simulink model "VOC7"  (R2022b)
settings: Solver=VariableStepAuto  StartTime=0.0  StopTime=2  RelTol=1e-3
libraries: spsIGBTDiodeLib x12, spsSeriesRLCBranchLib x7, eeRmsMeasurement x6, spsVoltageMeasurementLib x4, spsCurrentMeasurementLib x3, spsDCVoltageSourceLib x3, spspowerguiLib x1
settings Model: Creator=LEGION  LastModifiedBy=DoCongHieu
settings DebuggingCC: UnconnectedInputMsg=warning  UnconnectedOutputMsg=warning  UnconnectedLineMsg=warning
settings ModelReferenceCC: EnableRefExpFcnMdlSchedulingChecks=on
settings RTWCC: DLArmComputeVersion=19.05

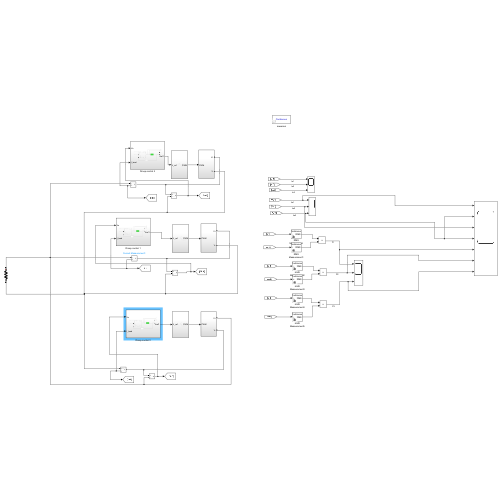
[thumbnail: Simulink's stored preview of the top-level diagram]
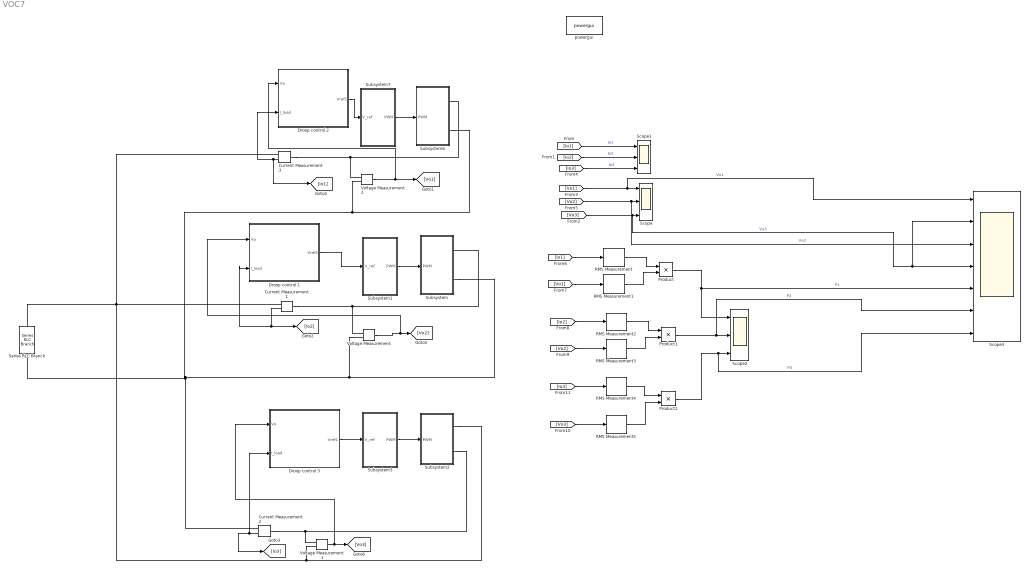
== system VOC7 ==
  Current Measurement1 : spsCurrentMeasurementLib/Current Measurement  PhasorSimulation=off  OutputType=Complex  PSBequivalent=0
  Current Measurement2 : spsCurrentMeasurementLib/Current Measurement  PhasorSimulation=off  OutputType=Complex  PSBequivalent=0
  Current Measurement3 : spsCurrentMeasurementLib/Current Measurement  PhasorSimulation=off  OutputType=Complex  PSBequivalent=0
  Droop control 1 : Subsystem
  Droop control 2 : Subsystem
  Droop control 3 : Subsystem
  Product : Product
  Product1 : Product
  Product2 : Product
  RMS Measurement{,1..5} (6 alike) : eeRmsMeasurement/RMS Measurement  LabelModeActiveChoice=Total  F=60  SpecifyHarmonics=off  K=[0 1 2]  Ts=0
      settings: LibrarySourceBlock=|
      | ee_sl_lib/Measurements/RMS
      | Measurement
  Scope : Scope  NumInputPorts=3
  Scope1 : Scope  NumInputPorts=3
  Scope2 : Scope  NumInputPorts=3
  Scope3 : Scope  NumInputPorts=7
  Series RLC Branch : spsSeriesRLCBranchLib/Series RLC Branch  LConnTagsString=__new0  RConnTagsString=__new0  BranchType=R  Resistance=10  Inductance=1e-3  SetiL0=off  InitialCurrent=0  Capacitance=1e-6  Setx0=off  InitialVoltage=0  Measurements=None
  Subsystem : Subsystem
  Subsystem1 : Subsystem
  Subsystem2 : Subsystem
  Subsystem3 : Subsystem
  Subsystem6 : Subsystem
  Subsystem7 : Subsystem
  Voltage Measurement : spsVoltageMeasurementLib/Voltage Measurement  PhasorSimulation=off  OutputType=Complex  PSBequivalent=0
  Voltage Measurement1 : spsVoltageMeasurementLib/Voltage Measurement  PhasorSimulation=off  OutputType=Complex  PSBequivalent=0
  Voltage Measurement2 : spsVoltageMeasurementLib/Voltage Measurement  PhasorSimulation=off  OutputType=Complex  PSBequivalent=0
  powergui : spspowerguiLib/powergui  Priority=1  SimulationMode=Continuous  SampleTime=5e-6  frequency=60  Iterations=50  frequencyindice=0  Pbase=100e6  ErrMax=1e-4  UnitsV=kV  UnitsW=MW  buscounter=0  FunctionMessages=off  echomessages=off  EnableUseOfTLC=off  CurrentSourceSwitches=off  DisableSnubberDevices=off  DisableRonSwitches=off  DisableVfSwitches=off  DisplayEquations=off  AutomaticDiscreteSolvers=off  SolverType=Tustin/Backward Euler (TBE)  Interpol=off  ExternalGateDelay=off  methode=off  Ts=100  x0status=blocks  SPID=on  SwTol=0  HookPort=off  NonlinearTolerance=1e-4  nMaxIteration=100  ContinueOnMaxIteration=off  RestoreLinks=warning  ResistiveCurrentMeasurement=off  Frange=[0:2:500]  Ylog=off  Xlog=on  ShowGrid=off  save=off  variable=ZData  structure=0  ZoomFFT=off  StartTime=0.0  cycles=1  DisplayStyle=1  fundamental=60  FreqAxis=off  MaxFrequency=1000  frequencyindicesteady=1  RmsSteady=1  display=off
  wires:
  Current Measurement1/1 -> [Io2], Droop control 1/2(I_load)
  [Io2] -> Scope1/2  "Io2"
  [Io1] -> Scope1/1  "Io1"
  Subsystem1/1(PWM) -> Subsystem/1(PWM)
  Subsystem3/1(PWM) -> Subsystem2/1("PWM ")
  RMS Measurement/1 -> Product/1
  RMS Measurement1/1 -> Product/2
  Voltage Measurement/1 -> Droop control 1/1(Vo), [Vo2]
  [Vo1] -> Scope3/1, Scope/1  "Vo1"
  [Vo2] -> Scope3/3, Scope/2  "Vo2"
  [Vo1] -> RMS Measurement1/1
  [Io1] -> RMS Measurement/1
  RMS Measurement3/1 -> Product1/2
  [Vo2] -> RMS Measurement3/1
  [Io2] -> RMS Measurement2/1
  RMS Measurement2/1 -> Product1/1
  Product/1 -> Scope2/1, Scope3/5  "P1"
  Product1/1 -> Scope3/6, Scope2/2  "P2"
  Subsystem7/1(PWM) -> Subsystem6/1(PWM)
  Current Measurement3/1 -> Droop control 2/2(I_load), [Io1]
  Voltage Measurement2/1 -> Droop control 2/1(Vo), [Vo1]
  RMS Measurement5/1 -> Product2/2
  RMS Measurement4/1 -> Product2/1
  Product2/1 -> Scope3/7, Scope2/3  "P3"
  [Vo3] -> Scope3/2, Scope3/4, Scope/3  "Vo3"
  [Io3] -> Scope1/3  "Io3"
  [Vo3] -> RMS Measurement5/1
  [Io3] -> RMS Measurement4/1
  Droop control 1/1(Vref1) -> Subsystem1/1(V_ref)
  Droop control 2/1(Vref1) -> Subsystem7/1(V_ref)
  Voltage Measurement1/1 -> Droop control 3/1(Vo), [Vo3]
  Current Measurement2/1 -> Droop control 3/2(I_load), [Io3]
  Droop control 3/1(Vref1) -> Subsystem3/1(V_ref)
  connections:
  Current Measurement1/LConn1 -- Voltage Measurement/LConn1 -- Subsystem/RConn1
  Series RLC Branch/LConn1 -- Voltage Measurement1/LConn2 -- Subsystem2/RConn1 -- Current Measurement3/RConn1 -- Current Measurement1/RConn1
  Subsystem6/RConn1 -- Current Measurement3/LConn1 -- Voltage Measurement2/LConn1
  Series RLC Branch/RConn1 -- Subsystem/RConn2 -- Voltage Measurement/LConn2 -- Subsystem6/RConn2 -- Voltage Measurement2/LConn2 -- Current Measurement2/RConn1
  Subsystem2/RConn2 -- Voltage Measurement1/LConn1 -- Current Measurement2/LConn1

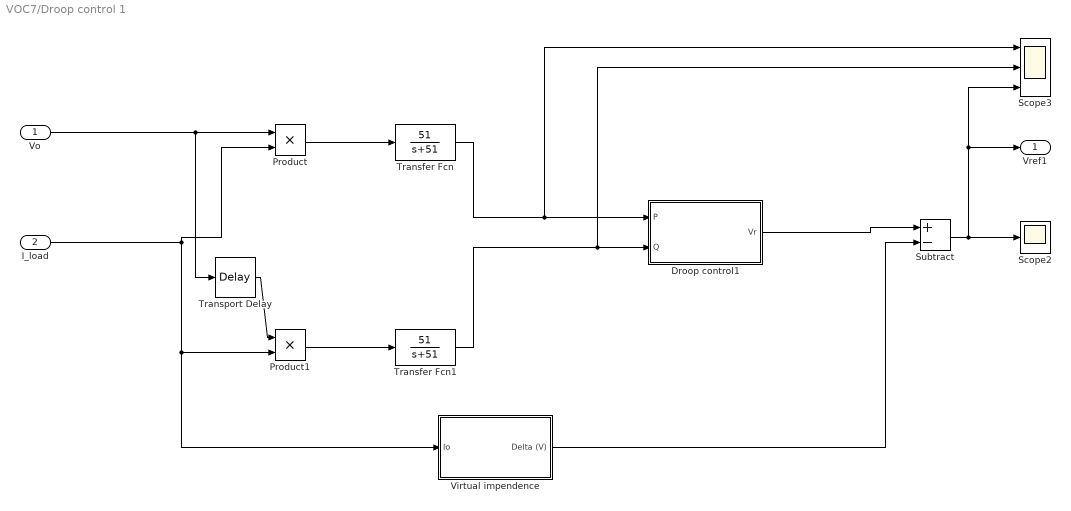
== system VOC7/Droop control 1 ==
  Vo : Inport
  I_load : Inport  Port=2
  Droop control1 : Subsystem  mask{Mi=0.0081, Ni=7.85e-4, E_ref=200*1.1, f_ref=1.01*50, f=50}
      mask prompts: Mi "Vol.coefficient"; Ni "Fre.coefficent"; E_ref "Ref.voltage"; f_ref "Ref.frequency"; f "Fund.frequency"
  Product : Product
  Product1 : Product
  Scope2 : Scope
  Scope3 : Scope  NumInputPorts=3
  Subtract : Sum  Inputs=+-
  Transfer Fcn : TransferFcn  Numerator=[51]  Denominator=[1 51]
  Transfer Fcn1 : TransferFcn  Numerator=[51]  Denominator=[1 51]
  Transport Delay : TransportDelay  DelayTime=0.02/4
  Virtual impendence : Subsystem  mask{fp=150, Rv=0, Lv=2e-3}
      mask prompts: fp "Cutoff Fred"
  Vref1 : Outport
  wires:
  Vo/1 -> Product/1, Transport Delay/1
  I_load/1 -> Product/2, Virtual impendence/1(Io), Product1/2
  Transport Delay/1 -> Product1/1
  Product/1 -> Transfer Fcn/1
  Product1/1 -> Transfer Fcn1/1
  Virtual impendence/1(Delta (V)) -> Subtract/2
  Transfer Fcn1/1 -> Scope3/2, Droop control1/2(Q)
  Droop control1/1(Vr) -> Subtract/1
  Transfer Fcn/1 -> Scope3/1, Droop control1/1(P)
  Subtract/1 -> Scope2/1, Scope3/3, Vref1/1

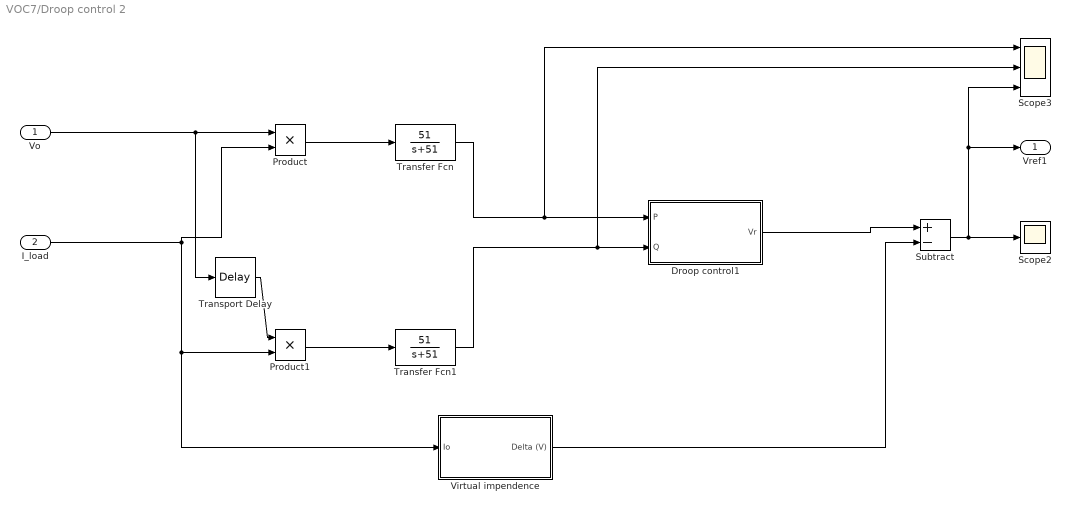
== system VOC7/Droop control 2 ==
  Vo : Inport
  I_load : Inport  Port=2
  Droop control1 : Subsystem  mask{Mi=0.0081, Ni=7.85e-4, E_ref=200*1.1, f_ref=1.01*50, f=50}
      mask prompts: Mi "Vol.coefficient"; Ni "Fre.coefficent"; E_ref "Ref.voltage"; f_ref "Ref.frequency"; f "Fund.frequency"
  Product : Product
  Product1 : Product
  Scope2 : Scope
  Scope3 : Scope  NumInputPorts=3
  Subtract : Sum  Inputs=+-
  Transfer Fcn : TransferFcn  Numerator=[51]  Denominator=[1 51]
  Transfer Fcn1 : TransferFcn  Numerator=[51]  Denominator=[1 51]
  Transport Delay : TransportDelay  DelayTime=0.02/4
  Virtual impendence : Subsystem  mask{fp=150, Rv=0, Lv=2e-3}
      mask prompts: fp "Cutoff Fred"
  Vref1 : Outport
  wires:
  Vo/1 -> Product/1, Transport Delay/1
  I_load/1 -> Product/2, Virtual impendence/1(Io), Product1/2
  Transport Delay/1 -> Product1/1
  Product/1 -> Transfer Fcn/1
  Product1/1 -> Transfer Fcn1/1
  Virtual impendence/1(Delta (V)) -> Subtract/2
  Transfer Fcn1/1 -> Scope3/2, Droop control1/2(Q)
  Droop control1/1(Vr) -> Subtract/1
  Transfer Fcn/1 -> Scope3/1, Droop control1/1(P)
  Subtract/1 -> Scope2/1, Scope3/3, Vref1/1

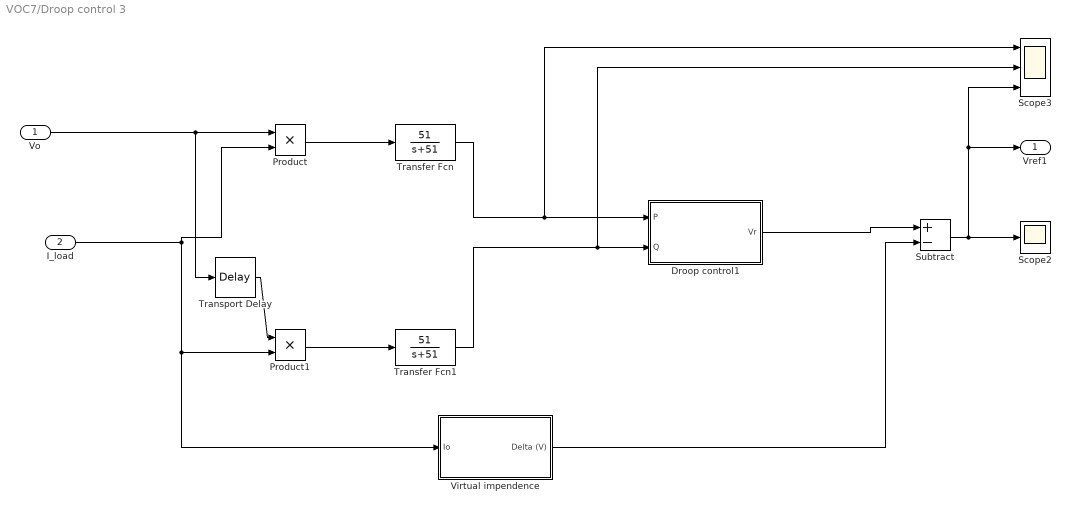
== system VOC7/Droop control 3 ==
  Vo : Inport
  I_load : Inport  Port=2
  Droop control1 : Subsystem  mask{Mi=0.0081, Ni=7.85e-4, E_ref=200*1.1, f_ref=1.01*50, f=50}
      mask prompts: Mi "Vol.coefficient"; Ni "Fre.coefficent"; E_ref "Ref.voltage"; f_ref "Ref.frequency"; f "Fund.frequency"
  Product : Product
  Product1 : Product
  Scope2 : Scope
  Scope3 : Scope  NumInputPorts=3
  Subtract : Sum  Inputs=+-
  Transfer Fcn : TransferFcn  Numerator=[51]  Denominator=[1 51]
  Transfer Fcn1 : TransferFcn  Numerator=[51]  Denominator=[1 51]
  Transport Delay : TransportDelay  DelayTime=0.02/4
  Virtual impendence : Subsystem  mask{fp=150, Rv=0, Lv=2e-3}
      mask prompts: fp "Cutoff Fred"
  Vref1 : Outport
  wires:
  Vo/1 -> Product/1, Transport Delay/1
  I_load/1 -> Product/2, Virtual impendence/1(Io), Product1/2
  Transport Delay/1 -> Product1/1
  Product/1 -> Transfer Fcn/1
  Product1/1 -> Transfer Fcn1/1
  Virtual impendence/1(Delta (V)) -> Subtract/2
  Transfer Fcn1/1 -> Scope3/2, Droop control1/2(Q)
  Droop control1/1(Vr) -> Subtract/1
  Transfer Fcn/1 -> Scope3/1, Droop control1/1(P)
  Subtract/1 -> Scope2/1, Scope3/3, Vref1/1

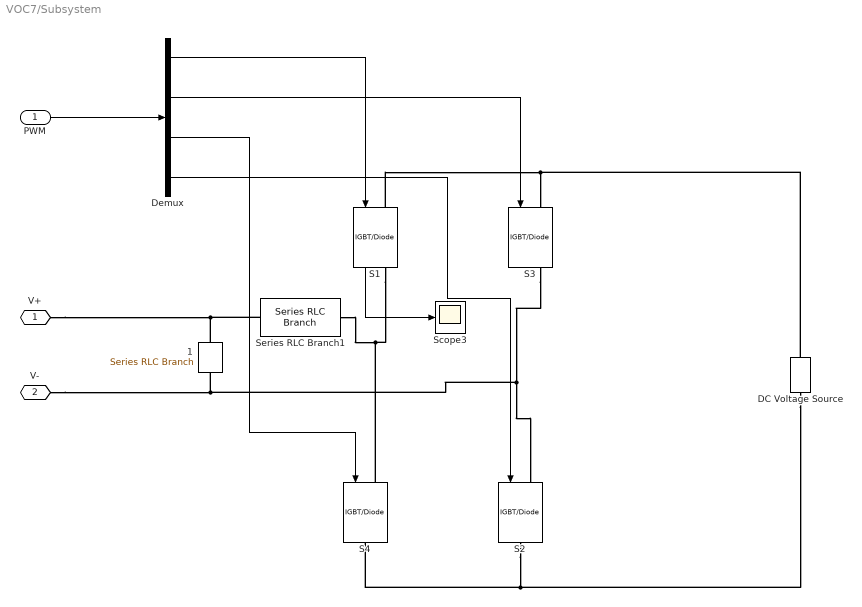
== system VOC7/Subsystem ==
  PWM : Inport
  " 1" : spsSeriesRLCBranchLib/Series RLC Branch  LConnTagsString=__new0  RConnTagsString=__new0  BranchType=C  Resistance=1  Inductance=1e-3  SetiL0=off  InitialCurrent=0  Capacitance=0.00009044  Setx0=off  InitialVoltage=0  Measurements=None
  DC Voltage Source : spsDCVoltageSourceLib/DC Voltage Source  Amplitude=350  Measurements=None
  Demux : Demux
  S1 : spsIGBTDiodeLib/IGBT//Diode  Ron=1e-3  Rs=1e5  Cs=inf  Measurements=on
  S2 : spsIGBTDiodeLib/IGBT//Diode  Ron=1e-3  Rs=1e5  Cs=inf  Measurements=off
  S3 : spsIGBTDiodeLib/IGBT//Diode  Ron=1e-3  Rs=1e5  Cs=inf  Measurements=on
  S4 : spsIGBTDiodeLib/IGBT//Diode  Ron=1e-3  Rs=1e5  Cs=inf  Measurements=off
  Scope3 : Scope
  Series RLC Branch1 : spsSeriesRLCBranchLib/Series RLC Branch  LConnTagsString=__new0  RConnTagsString=__new0  BranchType=L  Resistance=1  Inductance=0.0002882  SetiL0=off  InitialCurrent=0  Capacitance=1e-6  Setx0=off  InitialVoltage=0  Measurements=None
  V+ : PMIOPort  Side=Right
  V- : PMIOPort  Port=2  Side=Right
  wires:
  Demux/1 -> S1/1
  Demux/2 -> S3/1
  Demux/3 -> S4/1
  Demux/4 -> S2/1
  S1/1 -> Scope3/1
  PWM/1 -> Demux/1
  connections:
  DC Voltage Source/RConn1 -- S3/LConn1 -- S1/LConn1
  DC Voltage Source/LConn1 -- S4/RConn1 -- S2/RConn1
  S2/LConn1 -- S3/RConn1 -- V-/RConn1 -- " 1"/RConn1
  S4/LConn1 -- Series RLC Branch1/RConn1 -- S1/RConn1
  V+/RConn1 -- Series RLC Branch1/LConn1 -- " 1"/LConn1

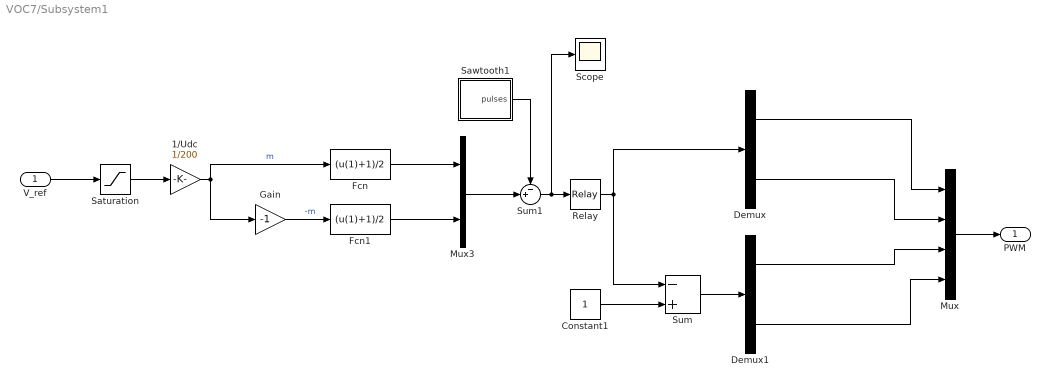
== system VOC7/Subsystem1 ==
  V_ref : Inport
  1/Udc : Gain  Gain=1/200
  Constant1 : Constant
  Demux : Demux  Outputs=2
  Demux1 : Demux  Outputs=2
  Fcn : Fcn  Expr=(u(1)+1)/2
  Fcn1 : Fcn  Expr=(u(1)+1)/2
  Gain : Gain  Gain=-1
  Mux : Mux
  Mux3 : Mux  Inputs=2
  Relay : Relay
  Saturation : Saturate  UpperLimit=310  LowerLimit=-310
  Sawtooth1 : Subsystem
  Scope : Scope
  Sum : Sum  Inputs=-+
  Sum1 : Sum  Inputs=-+|  InputSameDT=on  SaturateOnIntegerOverflow=on  OutDataTypeStr=Inherit: Same as first input
  PWM : Outport
  wires:
  Relay/1 -> Demux/1, Sum/1
  Saturation/1 -> 1/Udc/1
  Demux1/1 -> Mux/3
  Sum/1 -> Demux1/1
  Fcn1/1 -> Mux3/2
  Gain/1 -> Fcn1/1  "-m"
  Constant1/1 -> Sum/2
  1/Udc/1 -> Fcn/1, Gain/1  "m"
  Sum1/1 -> Scope/1, Relay/1
  Demux/2 -> Mux/2
  Demux1/2 -> Mux/4
  Demux/1 -> Mux/1
  Sawtooth1/1(pulses) -> Sum1/1
  Mux3/1 -> Sum1/2
  Fcn/1 -> Mux3/1
  V_ref/1 -> Saturation/1
  Mux/1 -> PWM/1

== system VOC7/Subsystem2 ==
  "PWM " : Inport
  " 1" : spsSeriesRLCBranchLib/Series RLC Branch  LConnTagsString=__new0  RConnTagsString=__new0  BranchType=C  Resistance=1  Inductance=1e-3  SetiL0=off  InitialCurrent=0  Capacitance=0.00009044  Setx0=off  InitialVoltage=0  Measurements=None
  DC Voltage Source : spsDCVoltageSourceLib/DC Voltage Source  Amplitude=350  Measurements=None
  Demux : Demux
  S1 : spsIGBTDiodeLib/IGBT//Diode  Ron=1e-3  Rs=1e5  Cs=inf  Measurements=on
  S2 : spsIGBTDiodeLib/IGBT//Diode  Ron=1e-3  Rs=1e5  Cs=inf  Measurements=off
  S3 : spsIGBTDiodeLib/IGBT//Diode  Ron=1e-3  Rs=1e5  Cs=inf  Measurements=on
  S4 : spsIGBTDiodeLib/IGBT//Diode  Ron=1e-3  Rs=1e5  Cs=inf  Measurements=off
  Series RLC Branch1 : spsSeriesRLCBranchLib/Series RLC Branch  LConnTagsString=__new0  RConnTagsString=__new0  BranchType=L  Resistance=1  Inductance=0.0002882  SetiL0=off  InitialCurrent=0  Capacitance=1e-6  Setx0=off  InitialVoltage=0  Measurements=None
  V+ : PMIOPort  Side=Right
  V- : PMIOPort  Port=2  Side=Right
  wires:
  Demux/1 -> S1/1
  Demux/2 -> S3/1
  Demux/3 -> S4/1
  Demux/4 -> S2/1
  "PWM "/1 -> Demux/1
  connections:
  DC Voltage Source/RConn1 -- S1/LConn1 -- S3/LConn1
  DC Voltage Source/LConn1 -- S4/RConn1 -- S2/RConn1
  S3/RConn1 -- V-/RConn1 -- " 1"/RConn1 -- S2/LConn1
  S4/LConn1 -- S1/RConn1 -- Series RLC Branch1/RConn1
  Series RLC Branch1/LConn1 -- V+/RConn1 -- " 1"/LConn1

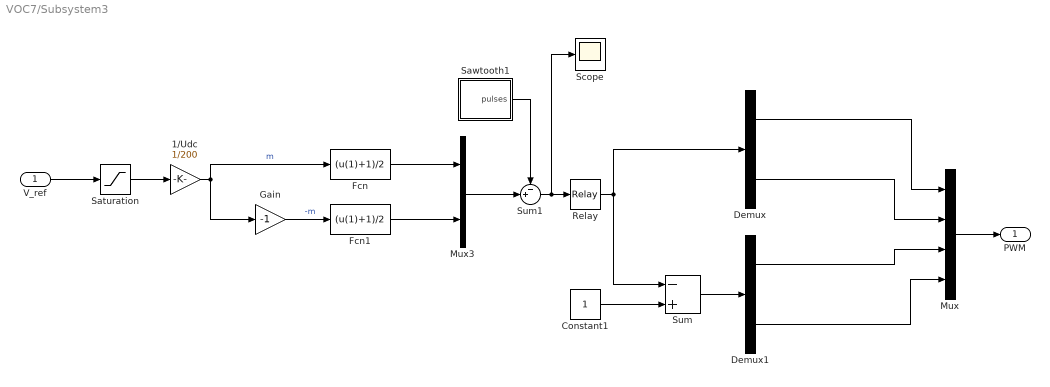
== system VOC7/Subsystem3 ==
  V_ref : Inport
  1/Udc : Gain  Gain=1/200
  Constant1 : Constant
  Demux : Demux  Outputs=2
  Demux1 : Demux  Outputs=2
  Fcn : Fcn  Expr=(u(1)+1)/2
  Fcn1 : Fcn  Expr=(u(1)+1)/2
  Gain : Gain  Gain=-1
  Mux : Mux
  Mux3 : Mux  Inputs=2
  Relay : Relay
  Saturation : Saturate  UpperLimit=310  LowerLimit=-310
  Sawtooth1 : Subsystem
  Scope : Scope
  Sum : Sum  Inputs=-+
  Sum1 : Sum  Inputs=-+|  InputSameDT=on  SaturateOnIntegerOverflow=on  OutDataTypeStr=Inherit: Same as first input
  PWM : Outport
  wires:
  Relay/1 -> Demux/1, Sum/1
  Saturation/1 -> 1/Udc/1
  Demux1/1 -> Mux/3
  Sum/1 -> Demux1/1
  Fcn1/1 -> Mux3/2
  Gain/1 -> Fcn1/1  "-m"
  Constant1/1 -> Sum/2
  1/Udc/1 -> Fcn/1, Gain/1  "m"
  Sum1/1 -> Scope/1, Relay/1
  Demux/2 -> Mux/2
  Demux1/2 -> Mux/4
  Demux/1 -> Mux/1
  Sawtooth1/1(pulses) -> Sum1/1
  Mux3/1 -> Sum1/2
  Fcn/1 -> Mux3/1
  V_ref/1 -> Saturation/1
  Mux/1 -> PWM/1

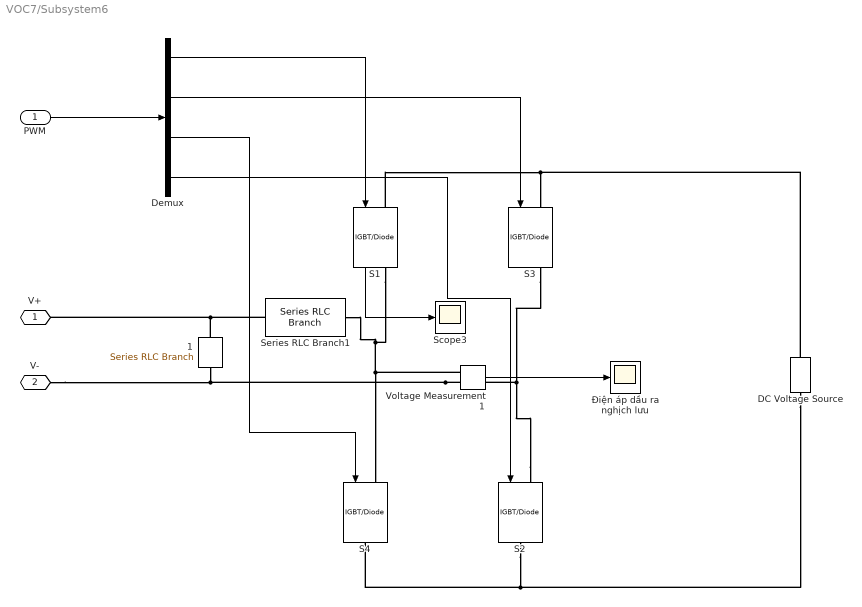
== system VOC7/Subsystem6 ==
  PWM : Inport
  " 1" : spsSeriesRLCBranchLib/Series RLC Branch  LConnTagsString=__new0  RConnTagsString=__new0  BranchType=C  Resistance=1  Inductance=1e-3  SetiL0=off  InitialCurrent=0  Capacitance=0.00009044  Setx0=off  InitialVoltage=0  Measurements=None
  DC Voltage Source : spsDCVoltageSourceLib/DC Voltage Source  Amplitude=350  Measurements=None
  Demux : Demux
  S1 : spsIGBTDiodeLib/IGBT//Diode  Ron=1e-3  Rs=1e5  Cs=inf  Measurements=on
  S2 : spsIGBTDiodeLib/IGBT//Diode  Ron=1e-3  Rs=1e5  Cs=inf  Measurements=off
  S3 : spsIGBTDiodeLib/IGBT//Diode  Ron=1e-3  Rs=1e5  Cs=inf  Measurements=on
  S4 : spsIGBTDiodeLib/IGBT//Diode  Ron=1e-3  Rs=1e5  Cs=inf  Measurements=off
  Scope3 : Scope
  Series RLC Branch1 : spsSeriesRLCBranchLib/Series RLC Branch  LConnTagsString=__new0  RConnTagsString=__new0  BranchType=L  Resistance=1  Inductance=0.0002882  SetiL0=off  InitialCurrent=0  Capacitance=1e-6  Setx0=off  InitialVoltage=0  Measurements=None
  Voltage Measurement1 : spsVoltageMeasurementLib/Voltage Measurement  PhasorSimulation=off  OutputType=Complex  PSBequivalent=0
  "Điện áp dầu ra nghịch lưu " : Scope
  V+ : PMIOPort  Side=Right
  V- : PMIOPort  Port=2  Side=Right
  wires:
  Demux/1 -> S1/1
  Demux/2 -> S3/1
  Demux/3 -> S4/1
  Demux/4 -> S2/1
  Voltage Measurement1/1 -> "Điện áp dầu ra nghịch lưu "/1
  S1/1 -> Scope3/1
  PWM/1 -> Demux/1
  connections:
  DC Voltage Source/RConn1 -- S3/LConn1 -- S1/LConn1
  DC Voltage Source/LConn1 -- S4/RConn1 -- S2/RConn1
  S2/LConn1 -- S3/RConn1 -- Voltage Measurement1/LConn2 -- " 1"/RConn1 -- V-/RConn1
  Voltage Measurement1/LConn1 -- S4/LConn1 -- Series RLC Branch1/RConn1 -- S1/RConn1
  V+/RConn1 -- Series RLC Branch1/LConn1 -- " 1"/LConn1

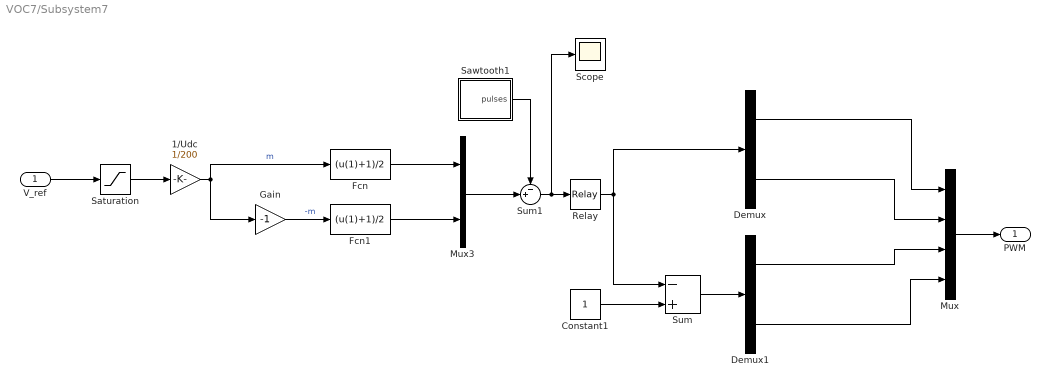
== system VOC7/Subsystem7 ==
  V_ref : Inport
  1/Udc : Gain  Gain=1/200
  Constant1 : Constant
  Demux : Demux  Outputs=2
  Demux1 : Demux  Outputs=2
  Fcn : Fcn  Expr=(u(1)+1)/2
  Fcn1 : Fcn  Expr=(u(1)+1)/2
  Gain : Gain  Gain=-1
  Mux : Mux
  Mux3 : Mux  Inputs=2
  Relay : Relay
  Saturation : Saturate  UpperLimit=310  LowerLimit=-310
  Sawtooth1 : Subsystem
  Scope : Scope
  Sum : Sum  Inputs=-+
  Sum1 : Sum  Inputs=-+|  InputSameDT=on  SaturateOnIntegerOverflow=on  OutDataTypeStr=Inherit: Same as first input
  PWM : Outport
  wires:
  Relay/1 -> Demux/1, Sum/1
  Saturation/1 -> 1/Udc/1
  Demux1/1 -> Mux/3
  Sum/1 -> Demux1/1
  Fcn1/1 -> Mux3/2
  Gain/1 -> Fcn1/1  "-m"
  Constant1/1 -> Sum/2
  1/Udc/1 -> Fcn/1, Gain/1  "m"
  Sum1/1 -> Scope/1, Relay/1
  Demux/2 -> Mux/2
  Demux1/2 -> Mux/4
  Demux/1 -> Mux/1
  Sawtooth1/1(pulses) -> Sum1/1
  Mux3/1 -> Sum1/2
  Fcn/1 -> Mux3/1
  V_ref/1 -> Saturation/1
  Mux/1 -> PWM/1

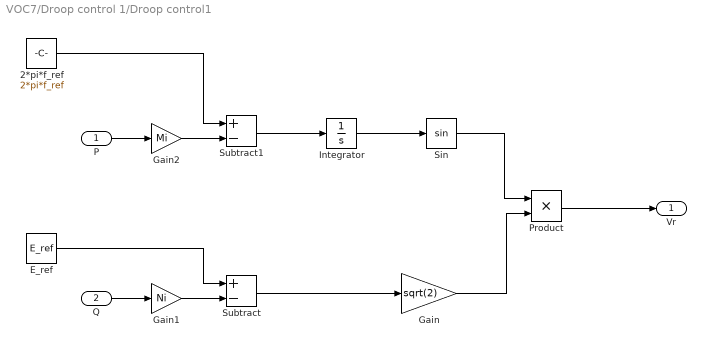
== system VOC7/Droop control 1/Droop control1 ==
  P : Inport
  Q : Inport  Port=2
  2*pi*f_ref : Constant  Value=2*pi*f_ref
  E_ref : Constant  Value=E_ref
  Gain : Gain  Gain=sqrt(2)
  Gain1 : Gain  Gain=Ni
  Gain2 : Gain  Gain=Mi
  Integrator : Integrator
  Product : Product
  Sin : Trigonometry
  Subtract : Sum  Inputs=+-
  Subtract1 : Sum  Inputs=+-
  Vr : Outport
  wires:
  Gain2/1 -> Subtract1/2
  2*pi*f_ref/1 -> Subtract1/1
  Integrator/1 -> Sin/1
  Subtract/1 -> Gain/1
  Subtract1/1 -> Integrator/1
  Gain/1 -> Product/2
  Sin/1 -> Product/1
  Gain1/1 -> Subtract/2
  E_ref/1 -> Subtract/1
  P/1 -> Gain2/1
  Q/1 -> Gain1/1
  Product/1 -> Vr/1

== system VOC7/Droop control 1/Virtual impendence ==
  Io : Inport
  Add : Sum
  Gain : Gain  Gain=Lv
  Gain1 : Gain  Gain=Rv
  Transfer Fcn : TransferFcn  Numerator=[2*pi*fp 0]  Denominator=[1 2*pi*fp]
  Delta (V) : Outport
  wires:
  Transfer Fcn/1 -> Gain/1
  Io/1 -> Gain1/1, Transfer Fcn/1
  Gain/1 -> Add/1
  Gain1/1 -> Add/2
  Add/1 -> Delta (V)/1

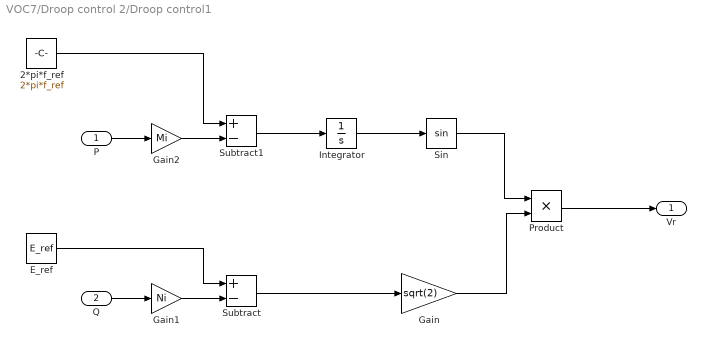
== system VOC7/Droop control 2/Droop control1 ==
  P : Inport
  Q : Inport  Port=2
  2*pi*f_ref : Constant  Value=2*pi*f_ref
  E_ref : Constant  Value=E_ref
  Gain : Gain  Gain=sqrt(2)
  Gain1 : Gain  Gain=Ni
  Gain2 : Gain  Gain=Mi
  Integrator : Integrator
  Product : Product
  Sin : Trigonometry
  Subtract : Sum  Inputs=+-
  Subtract1 : Sum  Inputs=+-
  Vr : Outport
  wires:
  Gain2/1 -> Subtract1/2
  2*pi*f_ref/1 -> Subtract1/1
  Integrator/1 -> Sin/1
  Subtract/1 -> Gain/1
  Subtract1/1 -> Integrator/1
  Gain/1 -> Product/2
  Sin/1 -> Product/1
  Gain1/1 -> Subtract/2
  E_ref/1 -> Subtract/1
  P/1 -> Gain2/1
  Q/1 -> Gain1/1
  Product/1 -> Vr/1

== system VOC7/Droop control 2/Virtual impendence ==
  Io : Inport
  Add : Sum
  Gain : Gain  Gain=Lv
  Gain1 : Gain  Gain=Rv
  Transfer Fcn : TransferFcn  Numerator=[2*pi*fp 0]  Denominator=[1 2*pi*fp]
  Delta (V) : Outport
  wires:
  Transfer Fcn/1 -> Gain/1
  Io/1 -> Gain1/1, Transfer Fcn/1
  Gain/1 -> Add/1
  Gain1/1 -> Add/2
  Add/1 -> Delta (V)/1

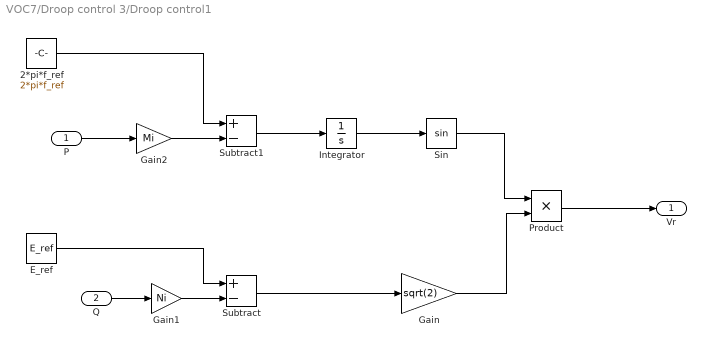
== system VOC7/Droop control 3/Droop control1 ==
  P : Inport
  Q : Inport  Port=2
  2*pi*f_ref : Constant  Value=2*pi*f_ref
  E_ref : Constant  Value=E_ref
  Gain : Gain  Gain=sqrt(2)
  Gain1 : Gain  Gain=Ni
  Gain2 : Gain  Gain=Mi
  Integrator : Integrator
  Product : Product
  Sin : Trigonometry
  Subtract : Sum  Inputs=+-
  Subtract1 : Sum  Inputs=+-
  Vr : Outport
  wires:
  Gain2/1 -> Subtract1/2
  2*pi*f_ref/1 -> Subtract1/1
  Integrator/1 -> Sin/1
  Subtract/1 -> Gain/1
  Subtract1/1 -> Integrator/1
  Gain/1 -> Product/2
  Sin/1 -> Product/1
  Gain1/1 -> Subtract/2
  E_ref/1 -> Subtract/1
  P/1 -> Gain2/1
  Q/1 -> Gain1/1
  Product/1 -> Vr/1

== system VOC7/Droop control 3/Virtual impendence ==
  Io : Inport
  Add : Sum
  Gain : Gain  Gain=Lv
  Gain1 : Gain  Gain=Rv
  Transfer Fcn : TransferFcn  Numerator=[2*pi*fp 0]  Denominator=[1 2*pi*fp]
  Delta (V) : Outport
  wires:
  Transfer Fcn/1 -> Gain/1
  Io/1 -> Gain1/1, Transfer Fcn/1
  Gain/1 -> Add/1
  Gain1/1 -> Add/2
  Add/1 -> Delta (V)/1

== system VOC7/Subsystem1/Sawtooth1 ==
  Integrator : Integrator
  Pulse Generator : DiscretePulseGenerator  PulseType=Time based  Period=1/100000  PulseWidth=50
  Scope3 : Scope
  Sum1 : Sum  Inputs=-+|  InputSameDT=on  SaturateOnIntegerOverflow=on  OutDataTypeStr=Inherit: Same as first input
  modulation index1 : Gain  Gain=2*100000  SaturateOnIntegerOverflow=on  OutDataTypeStr=Inherit: Same as input  ParamDataTypeStr=Inherit: Same as input
  modulation index2 : Gain  Gain=2  SaturateOnIntegerOverflow=on  OutDataTypeStr=Inherit: Same as input  ParamDataTypeStr=Inherit: Same as input
  pi/1 : Constant
  pulses : Outport  VectorParamsAs1DForOutWhenUnconnected=off
  wires:
  Pulse Generator/1 -> modulation index2/1
  Integrator/1 -> modulation index1/1
  modulation index1/1 -> pulses/1, Scope3/1
  Sum1/1 -> Integrator/1
  modulation index2/1 -> Sum1/2
  pi/1/1 -> Sum1/1

== system VOC7/Subsystem3/Sawtooth1 ==
  Integrator : Integrator
  Pulse Generator : DiscretePulseGenerator  PulseType=Time based  Period=1/100000  PulseWidth=50
  Scope3 : Scope
  Sum1 : Sum  Inputs=-+|  InputSameDT=on  SaturateOnIntegerOverflow=on  OutDataTypeStr=Inherit: Same as first input
  modulation index1 : Gain  Gain=2*100000  SaturateOnIntegerOverflow=on  OutDataTypeStr=Inherit: Same as input  ParamDataTypeStr=Inherit: Same as input
  modulation index2 : Gain  Gain=2  SaturateOnIntegerOverflow=on  OutDataTypeStr=Inherit: Same as input  ParamDataTypeStr=Inherit: Same as input
  pi/1 : Constant
  pulses : Outport  VectorParamsAs1DForOutWhenUnconnected=off
  wires:
  Pulse Generator/1 -> modulation index2/1
  Integrator/1 -> modulation index1/1
  modulation index1/1 -> pulses/1, Scope3/1
  Sum1/1 -> Integrator/1
  modulation index2/1 -> Sum1/2
  pi/1/1 -> Sum1/1

== system VOC7/Subsystem7/Sawtooth1 ==
  Integrator : Integrator
  Pulse Generator : DiscretePulseGenerator  PulseType=Time based  Period=1/100000  PulseWidth=50
  Scope3 : Scope
  Sum1 : Sum  Inputs=-+|  InputSameDT=on  SaturateOnIntegerOverflow=on  OutDataTypeStr=Inherit: Same as first input
  modulation index1 : Gain  Gain=2*100000  SaturateOnIntegerOverflow=on  OutDataTypeStr=Inherit: Same as input  ParamDataTypeStr=Inherit: Same as input
  modulation index2 : Gain  Gain=2  SaturateOnIntegerOverflow=on  OutDataTypeStr=Inherit: Same as input  ParamDataTypeStr=Inherit: Same as input
  pi/1 : Constant
  pulses : Outport  VectorParamsAs1DForOutWhenUnconnected=off
  wires:
  Pulse Generator/1 -> modulation index2/1
  Integrator/1 -> modulation index1/1
  modulation index1/1 -> pulses/1, Scope3/1
  Sum1/1 -> Integrator/1
  modulation index2/1 -> Sum1/2
  pi/1/1 -> Sum1/1
